simulink model "comm_projectB"  (R2020b)
settings: Solver=VariableStepAuto  StartTime=0.0  StopTime=0.002  FixedStep=0.001  MaxStep=0.000002  MinStep=0.000001  RelTol=1e-3
values from neighbouring files (symbols this model uses):
  kf = 5000    [comm_projectA.m]
settings Model: Creator=acer  LastModifiedBy=khale

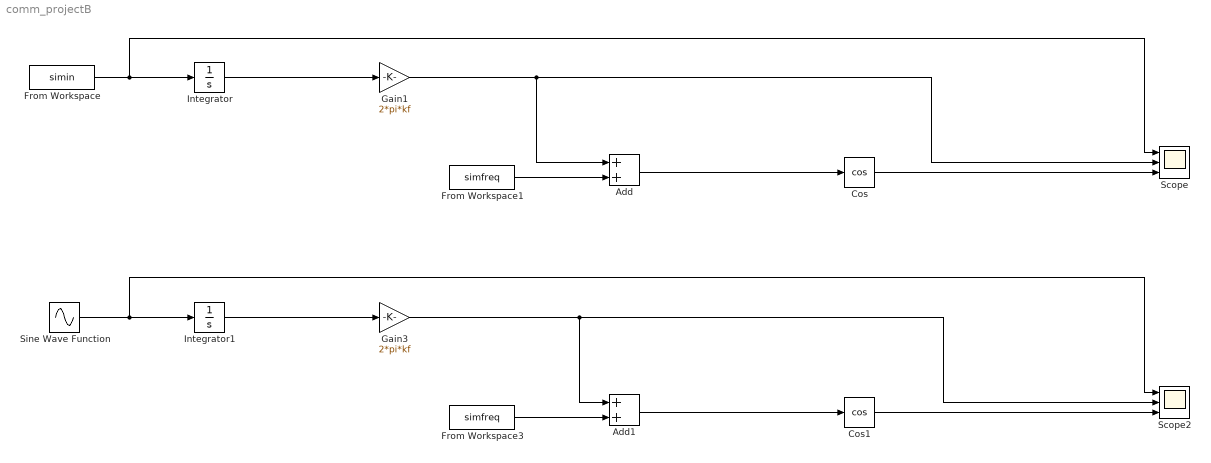
== system comm_projectB ==
  Add : Sum
  Add1 : Sum
  Cos : Trigonometry  Operator=cos
  Cos1 : Trigonometry  Operator=cos
  From Workspace : FromWorkspace  VariableName=simin
  From Workspace1 : FromWorkspace  VariableName=simfreq
  From Workspace3 : FromWorkspace  VariableName=simfreq
  Gain1 : Gain  Gain=2*pi*kf
  Gain3 : Gain  Gain=2*pi*kf
  Integrator : Integrator
  Integrator1 : Integrator
  Scope : Scope  NumInputPorts=3
  Scope2 : Scope  NumInputPorts=3
  Sine Wave Function : Sin  Amplitude=1.5  Frequency=2*pi*2000  SampleTime=0
  wires:
  Integrator/1 -> Gain1/1
  Gain1/1 -> Scope/2, Add/1
  From Workspace1/1 -> Add/2
  Add/1 -> Cos/1
  Cos/1 -> Scope/3
  From Workspace/1 -> Scope/1, Integrator/1
  Sine Wave Function/1 -> Scope2/1, Integrator1/1
  Gain3/1 -> Scope2/2, Add1/1
  Integrator1/1 -> Gain3/1
  From Workspace3/1 -> Add1/2
  Add1/1 -> Cos1/1
  Cos1/1 -> Scope2/3
